simulink model "IterationExample"  (R2020b)
settings: Solver=FixedStepDiscrete  StartTime=0.0  StopTime=10.0  RelTol=1e-3
settings Model: Creator=Lingf  LastModifiedBy=Lingf
settings DataIOCC: SaveOutput=off  SignalLogging=off  DSMLogging=off  SaveTime=off  ReturnWorkspaceOutputs=off

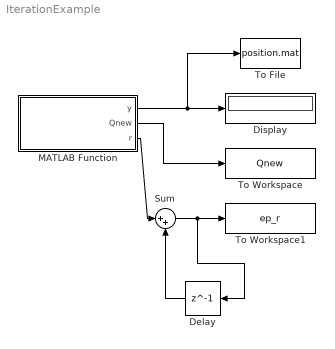
== system IterationExample ==
  Delay : Delay  DelayLength=1  InitialCondition=0
  Display : Display
  MATLAB Function : MATLAB Function  TreatAsAtomicUnit=on
  Sum : Sum  Inputs=|++
  To File : ToFile  Filename=position.mat
  To Workspace : ToWorkspace  VariableName=Qnew  SampleTime=-1
      settings: MaxDataPoints=1  Save2DSignal=2-D array (concatenate along first dimension)
  To Workspace1 : ToWorkspace  VariableName=ep_r  SampleTime=-1
      settings: MaxDataPoints=1  Save2DSignal=2-D array (concatenate along first dimension)
  wires:
  MATLAB Function/2(Qnew) -> To Workspace/1
  MATLAB Function/3(r) -> Sum/1
  Delay/1 -> Sum/2
  Sum/1 -> Delay/1, To Workspace1/1
  MATLAB Function/1(y) -> To File/1, Display/1

== matlab function IterationExample/MATLAB Function ==
  data: y output; Q parameter; Qnew output; r output
function [y,Qnew,r]= fcn(Q)
Qnew=Q*2;
r = Qnew(1,1,1,1,1,1);
y = Q(1,2,1,2,1,2);
